simulink subsystem "halfcar_subsystem"  (R2020b)
settings: Solver=VariableStepAuto  StartTime=0.0  StopTime=10.0  RelTol=1e-3
settings Model: Creator=Ricky  LastModifiedBy=Ricky

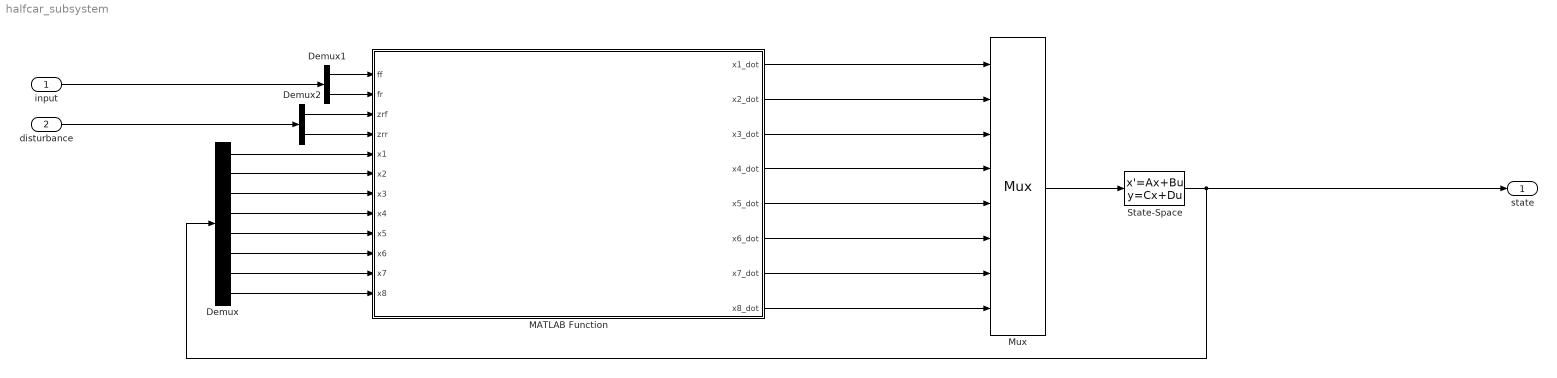
== system halfcar_subsystem ==
  input : Inport
  disturbance : Inport  Port=2
  Demux : Demux  Outputs=8
  Demux1 : Demux  Outputs=2
  Demux2 : Demux  Outputs=2
  MATLAB Function : MATLAB Function  TreatAsAtomicUnit=on
  Mux : Mux  Inputs=8
  State-Space : StateSpace  A=zeros(8)  B=eye(8)  C=eye(8)  D=zeros(8)  InitialCondition=0
  state : Outport
  wires:
  Demux/3 -> MATLAB Function/7(x3)
  MATLAB Function/1(x1_dot) -> Mux/1
  State-Space/1 -> Demux/1, state/1
  MATLAB Function/3(x3_dot) -> Mux/3
  disturbance/1 -> Demux2/1
  Mux/1 -> State-Space/1
  MATLAB Function/7(x7_dot) -> Mux/7
  MATLAB Function/8(x8_dot) -> Mux/8
  MATLAB Function/6(x6_dot) -> Mux/6
  Demux2/1 -> MATLAB Function/3(zrf)
  MATLAB Function/5(x5_dot) -> Mux/5
  Demux/6 -> MATLAB Function/10(x6)
  Demux/8 -> MATLAB Function/12(x8)
  MATLAB Function/2(x2_dot) -> Mux/2
  Demux1/2 -> MATLAB Function/2(fr)
  MATLAB Function/4(x4_dot) -> Mux/4
  Demux/1 -> MATLAB Function/5(x1)
  Demux1/1 -> MATLAB Function/1(ff)
  Demux2/2 -> MATLAB Function/4(zrr)
  input/1 -> Demux1/1
  Demux/5 -> MATLAB Function/9(x5)
  Demux/2 -> MATLAB Function/6(x2)
  Demux/4 -> MATLAB Function/8(x4)
  Demux/7 -> MATLAB Function/11(x7)

== matlab function halfcar_subsystem/MATLAB Function ==
  data: ff input; x1_dot output; fr input; zrf input; zrr input; x1 input; x2 input; x3 input; x4 input; x5 input; x6 input; x7 input; x8 input; x2_dot output; x3_dot output; x4_dot output; x5_dot output; x6_dot output; x7_dot output; x8_dot output
function [x1_dot,x2_dot,x3_dot,x4_dot,x5_dot,x6_dot,x7_dot,x8_dot] = fcn(ff,fr,zrf,zrr,x1,x2,x3,x4,x5,x6,x7,x8)

m_s = 879.35;
B_f = 1189;
B_r = 998;
K_f = 66793;
K_r = 18606;
K_tf = 201021;
K_tr = 201021;
m_uf = 43.76;
m_ur = 43.76;
J_y = 1283;
a = 1.5;
b = 1.5;

x1_dot = x2;
x2_dot = 1/m_s*(-(B_f+B_r)*x2+(a*B_f-b*B_r)*x4*cos(x3)-K_f*x5+B_f*x6-K_r*x7+B_r*x8+(ff+fr)+K_tf*zrf+K_tr*zrr);
x3_dot = x4;
x4_dot = 1/J_y*((a*B_f-b*B_r)*x2*cos(x3)-(a^2*B_f+b^2*B_r)*x4*cos(x3)^2+a*K_f*x5*cos(x3)-a*B_f*x6*cos(x3)-b*K_r*x7*cos(x3)+b*B_r*x8*cos(x3)+(a*ff+b*fr)*cos(x3)+K_tf*zrf+K_tr*zrr);
x5_dot = x2-a*x4*cos(x3)-x6;
x6_dot = 1/m_uf*(-K_tf*x1+B_f*x2+a*K_tf*sin(x3)-a*B_f*x4*cos(x3)+(K_f+K_tf)*x5-B_f*x6+K_tf*zrf-ff);
x7_dot = x2+b*x4*cos(x3)-x8;
x8_dot = 1/m_ur*(-K_tr*x1+B_r*x2-b*K_tr*sin(x3)-b*B_r*x4*cos(x3)+(K_r+K_tr)*x7-B_r*x8+K_tr*zrr-fr);
